simulink model "exc_sim"  (R2021a)
settings: Solver=VariableStepAuto  StartTime=0.0  StopTime=50  RelTol=1e-3
settings Model: Creator=davidrico  LastModifiedBy=davidrico

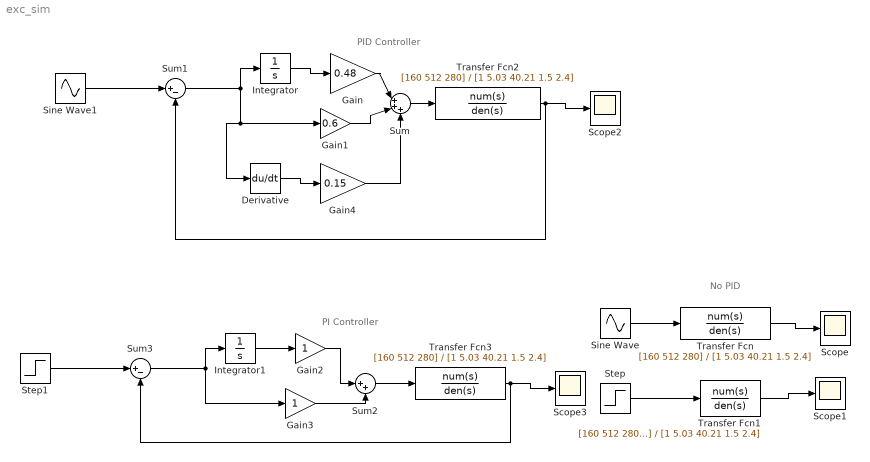
== system exc_sim ==
  note: No PID
  note: PID Controller
  note: PI Controller
  Derivative : Derivative
  Gain : Gain  Gain=0.48
  Gain1 : Gain  Gain=0.6
  Gain2 : Gain
  Gain3 : Gain
  Gain4 : Gain  Gain=0.15
  Integrator : Integrator
  Integrator1 : Integrator
  Scope{,1..3} (4 alike) : Scope
  Sine Wave : Sin  Frequency=pi  SampleTime=0
  Sine Wave1 : Sin  Frequency=2.5  SampleTime=0
  Step : Step  SampleTime=0
  Step1 : Step  SampleTime=0
  Sum : Sum  Inputs=|+++
  Sum1 : Sum  Inputs=|+-
  Sum2 : Sum  Inputs=|++
  Sum3 : Sum  Inputs=|+-
  Transfer Fcn{,1..3} (4 alike) : TransferFcn  Numerator=[160 512 280]  Denominator=[1 5.03 40.21 1.5 2.4]
  wires:
  Sine Wave/1 -> Transfer Fcn/1
  Transfer Fcn/1 -> Scope/1
  Step/1 -> Transfer Fcn1/1
  Transfer Fcn1/1 -> Scope1/1
  Transfer Fcn2/1 -> Sum1/2, Scope2/1
  Sum/1 -> Transfer Fcn2/1
  Sum1/1 -> Gain1/1, Derivative/1, Integrator/1
  Integrator/1 -> Gain/1
  Gain/1 -> Sum/1
  Gain1/1 -> Sum/2
  Sine Wave1/1 -> Sum1/1
  Gain3/1 -> Sum2/2
  Step1/1 -> Sum3/1
  Sum2/1 -> Transfer Fcn3/1
  Integrator1/1 -> Gain2/1
  Gain2/1 -> Sum2/1
  Transfer Fcn3/1 -> Sum3/2, Scope3/1
  Sum3/1 -> Gain3/1, Integrator1/1
  Derivative/1 -> Gain4/1
  Gain4/1 -> Sum/3
